simulink model "MDSC_PLL"  (R2018b)
settings: Solver=VariableStepAuto  StartTime=0.0  StopTime=10.0  RelTol=1e-3
libraries: simulink x1, powerlib_meascontrol x1, powerlib x1
(part 2 of 2)

== system MDSC_PLL/MDSC_n/MDSC_n/DSC_Beta/Delay 7/Sin 2*pi*hr//n. ==
  note: 2*pi*hr/n
  Constant : Constant  Value=2*pi*hr*7/n
  Trigonometric Function : Trigonometry
  sin : Outport
  wires:
  Trigonometric Function/1 -> sin/1
  Constant/1 -> Trigonometric Function/1

== system MDSC_PLL/MDSC_n/MDSC_n/DSC_Beta/Delay 8/Cos 2*pi*hr//n ==
  note: 2*pi*hr/n
  Constant : Constant  Value=2*pi*hr*8/n
  Trigonometric Function : Trigonometry  Operator=cos
  cos : Outport
  wires:
  Constant/1 -> Trigonometric Function/1
  Trigonometric Function/1 -> cos/1

== system MDSC_PLL/MDSC_n/MDSC_n/DSC_Beta/Delay 8/Sin 2*pi*hr//n. ==
  note: 2*pi*hr/n
  Constant : Constant  Value=2*pi*hr*8/n
  Trigonometric Function : Trigonometry
  sin : Outport
  wires:
  Constant/1 -> Trigonometric Function/1
  Trigonometric Function/1 -> sin/1

== system MDSC_PLL/MDSC_n/MDSC_n/DSC_Beta/Delay 9/Cos 2*pi*hr//n ==
  note: 2*pi*hr/n
  Constant : Constant  Value=2*pi*hr*9/n
  Trigonometric Function : Trigonometry  Operator=cos
  cos : Outport
  wires:
  Constant/1 -> Trigonometric Function/1
  Trigonometric Function/1 -> cos/1

== system MDSC_PLL/MDSC_n/MDSC_n/DSC_Beta/Delay 9/Sin 2*pi*hr//n. ==
  note: 2*pi*hr/n
  Constant : Constant  Value=2*pi*hr*9/n
  Trigonometric Function : Trigonometry
  sin : Outport
  wires:
  Constant/1 -> Trigonometric Function/1
  Trigonometric Function/1 -> sin/1

== system MDSC_PLL/MDSC_n/MDSC_n/DSC_alpha/Delay 1/Cos 2*pi*hr//n ==
  note: 2*pi*hr/n
  Constant : Constant  Value=2*pi*hr/n
  Trigonometric Function : Trigonometry  Operator=cos
  cos : Outport
  wires:
  Trigonometric Function/1 -> cos/1
  Constant/1 -> Trigonometric Function/1

== system MDSC_PLL/MDSC_n/MDSC_n/DSC_alpha/Delay 1/Sin 2*pi*hr//n. ==
  note: 2*pi*hr/n
  Constant : Constant  Value=2*pi*hr/n
  Trigonometric Function : Trigonometry
  sin : Outport
  wires:
  Trigonometric Function/1 -> sin/1
  Constant/1 -> Trigonometric Function/1

== system MDSC_PLL/MDSC_n/MDSC_n/DSC_alpha/Delay 10/Cos 2*pi*hr//n ==
  note: 2*pi*hr/n
  Constant : Constant  Value=2*pi*hr*10/n
  Trigonometric Function : Trigonometry  Operator=cos
  cos : Outport
  wires:
  Constant/1 -> Trigonometric Function/1
  Trigonometric Function/1 -> cos/1

== system MDSC_PLL/MDSC_n/MDSC_n/DSC_alpha/Delay 10/Sin 2*pi*hr//n. ==
  note: 2*pi*hr/n
  Constant : Constant  Value=2*pi*hr*10/n
  Trigonometric Function : Trigonometry
  sin : Outport
  wires:
  Constant/1 -> Trigonometric Function/1
  Trigonometric Function/1 -> sin/1

== system MDSC_PLL/MDSC_n/MDSC_n/DSC_alpha/Delay 11/Cos 2*pi*hr//n ==
  note: 2*pi*hr/n
  Constant : Constant  Value=2*pi*hr*11/n
  Trigonometric Function : Trigonometry  Operator=cos
  cos : Outport
  wires:
  Trigonometric Function/1 -> cos/1
  Constant/1 -> Trigonometric Function/1

== system MDSC_PLL/MDSC_n/MDSC_n/DSC_alpha/Delay 11/Sin 2*pi*hr//n. ==
  note: 2*pi*hr/n
  Constant : Constant  Value=2*pi*hr*11/n
  Trigonometric Function : Trigonometry
  sin : Outport
  wires:
  Trigonometric Function/1 -> sin/1
  Constant/1 -> Trigonometric Function/1

== system MDSC_PLL/MDSC_n/MDSC_n/DSC_alpha/Delay 12/Cos 2*pi*hr//n ==
  note: 2*pi*hr/n
  Constant : Constant  Value=2*pi*hr*12/n
  Trigonometric Function : Trigonometry  Operator=cos
  cos : Outport
  wires:
  Constant/1 -> Trigonometric Function/1
  Trigonometric Function/1 -> cos/1

== system MDSC_PLL/MDSC_n/MDSC_n/DSC_alpha/Delay 12/Sin 2*pi*hr//n. ==
  note: 2*pi*hr/n
  Constant : Constant  Value=2*pi*hr*12/n
  Trigonometric Function : Trigonometry
  sin : Outport
  wires:
  Constant/1 -> Trigonometric Function/1
  Trigonometric Function/1 -> sin/1

== system MDSC_PLL/MDSC_n/MDSC_n/DSC_alpha/Delay 13/Cos 2*pi*hr//n ==
  note: 2*pi*hr/n
  Constant : Constant  Value=2*pi*hr*13/n
  Trigonometric Function : Trigonometry  Operator=cos
  cos : Outport
  wires:
  Trigonometric Function/1 -> cos/1
  Constant/1 -> Trigonometric Function/1

== system MDSC_PLL/MDSC_n/MDSC_n/DSC_alpha/Delay 13/Sin 2*pi*hr//n. ==
  note: 2*pi*hr/n
  Constant : Constant  Value=2*pi*hr*13/n
  Trigonometric Function : Trigonometry
  sin : Outport
  wires:
  Trigonometric Function/1 -> sin/1
  Constant/1 -> Trigonometric Function/1

== system MDSC_PLL/MDSC_n/MDSC_n/DSC_alpha/Delay 14/Cos 2*pi*hr//n ==
  note: 2*pi*hr/n
  Constant : Constant  Value=2*pi*hr*14/n
  Trigonometric Function : Trigonometry  Operator=cos
  cos : Outport
  wires:
  Constant/1 -> Trigonometric Function/1
  Trigonometric Function/1 -> cos/1

== system MDSC_PLL/MDSC_n/MDSC_n/DSC_alpha/Delay 14/Sin 2*pi*hr//n. ==
  note: 2*pi*hr/n
  Constant : Constant  Value=2*pi*hr*14/n
  Trigonometric Function : Trigonometry
  sin : Outport
  wires:
  Constant/1 -> Trigonometric Function/1
  Trigonometric Function/1 -> sin/1

== system MDSC_PLL/MDSC_n/MDSC_n/DSC_alpha/Delay 2/Cos 2*pi*hr//n ==
  note: 2*pi*hr/n
  Constant : Constant  Value=2*pi*hr*2/n
  Trigonometric Function : Trigonometry  Operator=cos
  cos : Outport
  wires:
  Constant/1 -> Trigonometric Function/1
  Trigonometric Function/1 -> cos/1

== system MDSC_PLL/MDSC_n/MDSC_n/DSC_alpha/Delay 2/SIn 2*pi*hr//n. ==
  note: 2*pi*hr/n
  Constant : Constant  Value=2*pi*hr*2/n
  Trigonometric Function : Trigonometry
  sin : Outport
  wires:
  Constant/1 -> Trigonometric Function/1
  Trigonometric Function/1 -> sin/1

== system MDSC_PLL/MDSC_n/MDSC_n/DSC_alpha/Delay 3/Cos 2*pi*hr//n ==
  note: 2*pi*hr/n
  Constant : Constant  Value=2*pi*hr*3/n
  Trigonometric Function : Trigonometry  Operator=cos
  cos : Outport
  wires:
  Trigonometric Function/1 -> cos/1
  Constant/1 -> Trigonometric Function/1

== system MDSC_PLL/MDSC_n/MDSC_n/DSC_alpha/Delay 3/Sin 2*pi*hr//n. ==
  note: 2*pi*hr/n
  Constant : Constant  Value=2*pi*hr*3/n
  Trigonometric Function : Trigonometry
  sin : Outport
  wires:
  Trigonometric Function/1 -> sin/1
  Constant/1 -> Trigonometric Function/1

== system MDSC_PLL/MDSC_n/MDSC_n/DSC_alpha/Delay 4/Cos 2*pi*hr//n ==
  note: 2*pi*hr/n
  Constant : Constant  Value=2*pi*hr*4/n
  Trigonometric Function : Trigonometry  Operator=cos
  cos : Outport
  wires:
  Constant/1 -> Trigonometric Function/1
  Trigonometric Function/1 -> cos/1

== system MDSC_PLL/MDSC_n/MDSC_n/DSC_alpha/Delay 4/Sin 2*pi*hr//n. ==
  note: 2*pi*hr/n
  Constant : Constant  Value=2*pi*hr*4/n
  Trigonometric Function : Trigonometry
  sin : Outport
  wires:
  Constant/1 -> Trigonometric Function/1
  Trigonometric Function/1 -> sin/1

== system MDSC_PLL/MDSC_n/MDSC_n/DSC_alpha/Delay 5/Cos 2*pi*hr//n ==
  note: 2*pi*hr/n
  Constant : Constant  Value=2*pi*hr*5/n
  Trigonometric Function : Trigonometry  Operator=cos
  cos : Outport
  wires:
  Trigonometric Function/1 -> cos/1
  Constant/1 -> Trigonometric Function/1

== system MDSC_PLL/MDSC_n/MDSC_n/DSC_alpha/Delay 5/Sin 2*pi*hr//n. ==
  note: 2*pi*hr/n
  Constant : Constant  Value=2*pi*hr*5/n
  Trigonometric Function : Trigonometry
  sin : Outport
  wires:
  Trigonometric Function/1 -> sin/1
  Constant/1 -> Trigonometric Function/1

== system MDSC_PLL/MDSC_n/MDSC_n/DSC_alpha/Delay 6/Cos 2*pi*hr//n ==
  note: 2*pi*hr/n
  Constant : Constant  Value=2*pi*hr*6/n
  Trigonometric Function : Trigonometry  Operator=cos
  cos : Outport
  wires:
  Trigonometric Function/1 -> cos/1
  Constant/1 -> Trigonometric Function/1

== system MDSC_PLL/MDSC_n/MDSC_n/DSC_alpha/Delay 6/Sin 2*pi*hr//n. ==
  note: 2*pi*hr/n
  Constant : Constant  Value=2*pi*hr*6/n
  Trigonometric Function : Trigonometry
  sin : Outport
  wires:
  Trigonometric Function/1 -> sin/1
  Constant/1 -> Trigonometric Function/1

== system MDSC_PLL/MDSC_n/MDSC_n/DSC_alpha/Delay 7/Cos 2*pi*hr//n ==
  note: 2*pi*hr/n
  Constant : Constant  Value=2*pi*hr*7/n
  Trigonometric Function : Trigonometry  Operator=cos
  cos : Outport
  wires:
  Constant/1 -> Trigonometric Function/1
  Trigonometric Function/1 -> cos/1

== system MDSC_PLL/MDSC_n/MDSC_n/DSC_alpha/Delay 7/Sin 2*pi*hr//n. ==
  note: 2*pi*hr/n
  Constant : Constant  Value=2*pi*hr*7/n
  Trigonometric Function : Trigonometry
  sin : Outport
  wires:
  Constant/1 -> Trigonometric Function/1
  Trigonometric Function/1 -> sin/1

== system MDSC_PLL/MDSC_n/MDSC_n/DSC_alpha/Delay 8/Cos 2*pi*hr//n ==
  note: 2*pi*hr/n
  Constant : Constant  Value=2*pi*hr*8/n
  Trigonometric Function : Trigonometry  Operator=cos
  cos : Outport
  wires:
  Trigonometric Function/1 -> cos/1
  Constant/1 -> Trigonometric Function/1

== system MDSC_PLL/MDSC_n/MDSC_n/DSC_alpha/Delay 8/Sin 2*pi*hr//n. ==
  note: 2*pi*hr/n
  Constant : Constant  Value=2*pi*hr*8/n
  Trigonometric Function : Trigonometry
  sin : Outport
  wires:
  Trigonometric Function/1 -> sin/1
  Constant/1 -> Trigonometric Function/1

== system MDSC_PLL/MDSC_n/MDSC_n/DSC_alpha/Delay 9/Cos 2*pi*hr//n ==
  note: 2*pi*hr/n
  Constant : Constant  Value=2*pi*hr*9/n
  Trigonometric Function : Trigonometry  Operator=cos
  cos : Outport
  wires:
  Trigonometric Function/1 -> cos/1
  Constant/1 -> Trigonometric Function/1

== system MDSC_PLL/MDSC_n/MDSC_n/DSC_alpha/Delay 9/Sin 2*pi*hr//n. ==
  note: 2*pi*hr/n
  Constant : Constant  Value=2*pi*hr*9/n
  Trigonometric Function : Trigonometry
  sin : Outport
  wires:
  Trigonometric Function/1 -> sin/1
  Constant/1 -> Trigonometric Function/1
